simulink model "workingAquisition_demo"  (Simulink 7.0)
settings: Solver=ode14x  StartTime=0.0  StopTime=inf  FixedStep=0.01  RelTol=1e-3
undefined symbols (not defined in the file): Model_626, Sensoray
libraries: rtwinlib x3, simulink x1
settings Model: Creator=Student  LastModifiedBy=Student  SimulationMode=external
settings HardwareCC: ProdHWDeviceType=Generic->32-bit Real-Time Simulator  TargetHWDeviceType=32-bit Generic  ProdEqTarget=off
settings RTWCC: SystemTargetFile=rtwin.tlc  TemplateMakefile=rtwin.tmf  Description=Real-Time Windows Target  ProcessScript=rtwin_make_rtw_hook
settings RTWinTargetCC: GenFloatMathFcnCalls=ANSI_C  ModelReferenceCompliant=off  CompOptLevelCompliant=off  PortableWordSizes=off  CCOptimize=on

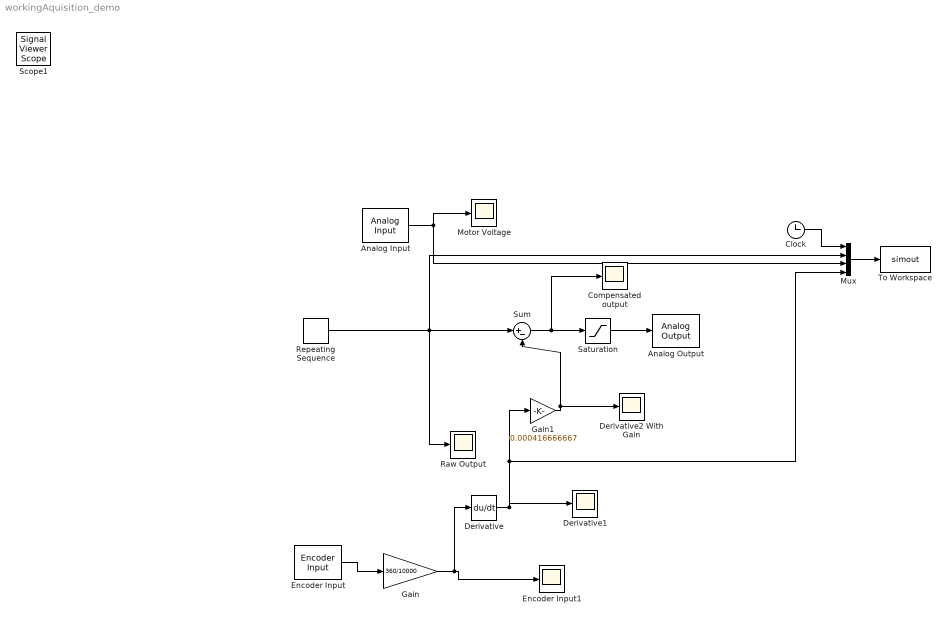
== system workingAquisition_demo ==
  Analog Input : rtwinlib/Analog Input  SampleTime=0.01  DrvName=Sensoray/Model_626  DrvAddress=4294967295  DrvOptions=zeros(1,0)  Channels=1  RangeMode=1  VoltRange=1  DataType=1
      settings: AttributesFormatString=Sensoray\nModel 626 [auto]
  Analog Output : rtwinlib/Analog Output  SampleTime=0.01  DrvName=Sensoray/Model_626  DrvAddress=4294967295  DrvOptions=zeros(1,0)  Channels=1  RangeMode=1  VoltRange=1  InitialValue=0  FinalValue=0
      settings: AttributesFormatString=Sensoray\nModel 626 [auto]
  Clock : Clock
      settings: Decimation=10
  Compensated output : Scope
      settings: YMin=-1  YMax=5.5  SaveName=position5  DataFormat=Array
  Derivative : Derivative
  Derivative1 : Scope
      settings: YMin=-1500  YMax=3000  SaveName=position3  DataFormat=Array
  Derivative2 With Gain : Scope
      settings: YMin=0  YMax=1.05  SaveName=position4  DataFormat=Array
  Encoder Input : rtwinlib/Encoder Input  SampleTime=0.01  DrvName=Sensoray/Model_626  DrvAddress=4294967295  DrvOptions=zeros(1,0)  Channels=[4]  QuadMode=3  IndexPulse=2  InputFilter=inf  DataType=1
      settings: AttributesFormatString=Sensoray\nModel 626 [auto]
  Encoder Input1 : Scope
      settings: YMin=-227000  YMax=-210000  SaveName=position  DataFormat=Array
  Gain : Gain  Gain=360/10000  ParameterDataType=sfix(16)  ParameterScaling=2^0  OutDataType=sfix(16)  OutScaling=2^0
  Gain1 : Gain  Gain=0.000416666667  ParameterDataType=sfix(16)  ParameterScaling=2^0  OutDataType=sfix(16)  OutScaling=2^0
  Motor Voltage : Scope
      settings: YMin=-7  YMax=7  SaveName=position1  DataFormat=Array
  Mux : Mux
  Raw Output : Scope
      settings: YMin=1.3  YMax=3  SaveName=position2  DataFormat=Array
  Repeating Sequence : simulink/Sources/Repeating Sequence  SystemSampleTime=-1  rep_seq_t=[0 3 6 9]  rep_seq_y=[1.37 3 3 1.37]
  Saturation : Saturate  UpperLimit=3  LowerLimit=0  OutDataType=sfix(16)  OutScaling=2^0
  Sum : Sum  Inputs=|+-  OutDataType=sfix(16)  OutScaling=2^0
  To Workspace : ToWorkspace  VariableName=simout  SampleTime=0.01  SaveFormat=Array
  Scope1 : SignalViewerScope  IOType=viewer  RefreshTime=0.035000
  wires:
  Encoder Input/1 -> Gain/1
  Gain/1 -> Encoder Input1/1, Derivative/1
  Analog Input/1 -> Motor Voltage/1, Mux/3
  Repeating Sequence/1 -> Sum/1, Mux/2, Raw Output/1
  Derivative/1 -> Derivative1/1, Gain1/1, Mux/4
  Gain1/1 -> Sum/2, Derivative2 With Gain/1
  Sum/1 -> Saturation/1, Compensated output/1
  Saturation/1 -> Analog Output/1
  Mux/1 -> To Workspace/1
  Clock/1 -> Mux/1
